simulink model "testWtAsset"  (R2012b)
settings: Solver=FixedStepDiscrete  StartTime=0.0  StopTime=86400  FixedStep=1  RelTol=1e-3
libraries: DiSC_ToolboxOpal_V11 x1
settings Model: Creator=Rasmus  LastModifiedBy=smartgrid
settings DataIOCC: SignalLoggingSaveFormat=ModelDataLogs
settings OptimizationCC: ExpressionDepthLimit=128
settings DebuggingCC: UnderspecifiedInitializationDetection=Simplified  MergeDetectMultiDrivingBlocksExec=error  MultiTaskDSMMsg=warning  MultiTaskCondExecSysMsg=none  StateNameClashWarn=none  StrictBusMsg=ErrorOnBusTreatedAsVector
settings RTWCC: IncludeERTFirstTime=on
settings CodeAppCC: CustomSymbolStrType=$N$R$M_T  InternalIdentifier=Shortened
settings GRTTargetCC: CodeReplacementLibrary=None  CPPClassGenCompliant=on

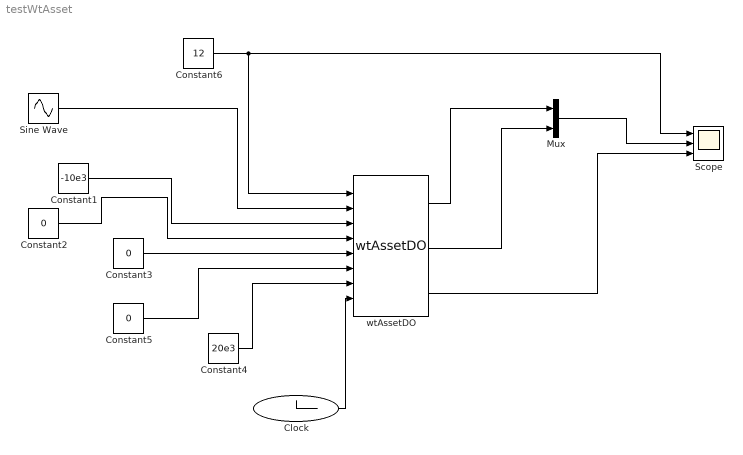
== system testWtAsset ==
  Clock : Clock
  Constant1 : Constant  Value=-10e3
  Constant2 : Constant  Value=0
  Constant3 : Constant  Value=0
  Constant4 : Constant  Value=20e3
  Constant5 : Constant  Value=0
  Constant6 : Constant  Value=12
  Mux : Mux  Inputs=2
  Scope : Scope  NumInputPorts=3
      settings: YMin=7~0~-100000  YMax=12~100000~100000  MaxDataPoints=50000
  Sine Wave : Sin  Amplitude=2000  Bias=20e3  Frequency=0.00008  SampleTime=0
  wtAssetDO : DiSC_ToolboxOpal_V11/wtAssetDO
  wires:
  Constant6/1 -> wtAssetDO/1, Scope/1
  Mux/1 -> Scope/2
  Sine Wave/1 -> wtAssetDO/2
  Constant1/1 -> wtAssetDO/3
  Constant2/1 -> wtAssetDO/4
  Constant3/1 -> wtAssetDO/5
  Constant5/1 -> wtAssetDO/6
  Constant4/1 -> wtAssetDO/7
  Clock/1 -> wtAssetDO/8
  wtAssetDO/1 -> Mux/1
  wtAssetDO/2 -> Mux/2
  wtAssetDO/3 -> Scope/3
